simulink model "lab5"  (R2023b)
settings: Solver=ode4  StartTime=0.0  StopTime=100.0  FixedStep=2^(-6)  RelTol=1e-3
settings Model: Creator=insomnia  LastModifiedBy=insomnia

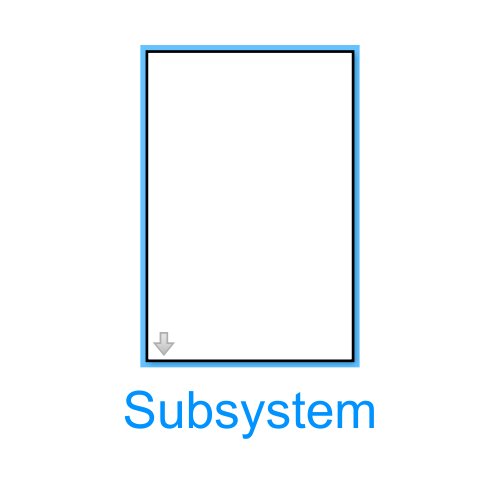
[thumbnail: Simulink's stored preview of the top-level diagram]
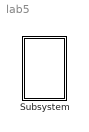
== system lab5 ==
  Subsystem : Subsystem  mask{g=9.81, l=2, m=3, k=5, r0=3, r1=1, th0=12, th1=6}

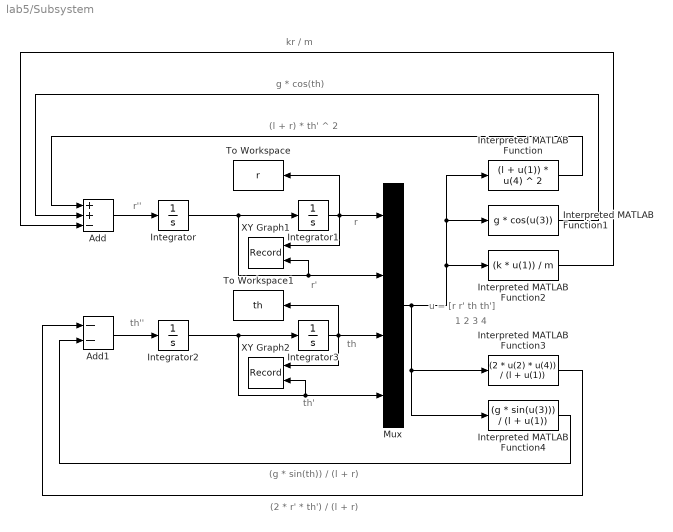
== system lab5/Subsystem ==
  note: (g * sin(th)) / (l + r)
  note: (2 * r' * th') / (l + r)
  note: th''
  note: r''
  note: kr / m
  note: g * cos(th)
  note: (l + r) * th' ^ 2
  note: th'
  note: th
  note: r'
  note: r
  note: 1 2 3 4
  note: u = [r r' th th']
  Add : Sum  Inputs=++-
  Add1 : Sum  Inputs=--
  Integrator : Integrator  InitialCondition=r1
  Integrator1 : Integrator  InitialCondition=r0
  Integrator2 : Integrator  InitialCondition=th1*pi/180
  Integrator3 : Integrator  InitialCondition=th0*pi/180
  Interpreted MATLAB Function : MATLABFcn  MATLABFcn=(l + u(1)) * u(4) ^ 2  OutputDimensions=1
  Interpreted MATLAB Function1 : MATLABFcn  MATLABFcn=g * cos(u(3))  OutputDimensions=1
  Interpreted MATLAB Function2 : MATLABFcn  MATLABFcn=(k * u(1)) / m  OutputDimensions=1
  Interpreted MATLAB Function3 : MATLABFcn  MATLABFcn=(2 * u(2) * u(4)) / (l + u(1))  OutputDimensions=1
  Interpreted MATLAB Function4 : MATLABFcn  MATLABFcn=(g * sin(u(3))) / (l + u(1))  OutputDimensions=1
  Mux : Mux
  To Workspace : ToWorkspace  VariableName=r  SampleTime=-1
  To Workspace1 : ToWorkspace  VariableName=th  SampleTime=-1
  XY Graph1 : Record  FileSettingsInternal="{\"entries\":[{\"content\":{\"excelSettings\":{\"content\":{},\"type\":\"Streamout.ExcelSettings\"}},\"type\":\"Streamout.FileSettingStorage\",\"uuid\":\"\"}],\"packageUris\":[\"http:\\/\\/schema.mathworks.com\\/mf0\\/streamout_blocks\\/R2020a\"],\"version\":\"1.0\"}"  Layout=[1 1]  SignalsInternal="{\"entries\":[{\"content\":{\"signals\":[{\"content\":{\"blockPath\":[],\"dimensions\":[1],\"domain\":\"\",\"lineColor\":\"#a2142f\",\"plots\":[ 1 ],\"port\":1,\"sid\":[\"\"],\"signalID\":1,\"signalName\":\"Integrator1\"},\"type\":\"RecordBlkView.Signal\",\"uuid\":\"\"},{\"content\":{\"blockPath\":[],\"dimensions\":[1],\"domain\":\"\",\"lineColor\":\"#139fff\",\"plots\":[ 1 ],\"port\":2,\"sid\":[\"\"],\"signalID\":2,\"signalName\":\"Integrator\"},\"type\":\"RecordBlkView.Signal\",\"uuid\":\"\"}]},\"type\":\"RecordBlkView.InputSignals\",\"uuid\":\"\"}],\"packageUris\":[\"http:\\/\\/schema.mathworks.com\\/mf0\\/streamout_blocks\\/R2020a\"],\"version\":\"1.0\"}"  VisualizationBindings="{\"xyplotplugin\":{\"info\":[{\"series\":[{\"bindingParametersList\":[{\"parameter\":\"X-Axis\",\"signalID\":1,\"signalName\":\"Integrator1\"},{\"parameter\":\"Y-Axis\",\"signalID\":2,\"signalName\":\"Integrator\"}],\"seriesID\":0}],\"subplotID\":1}]}}"  CompatibilityTag=XY
  XY Graph2 : Record  FileSettingsInternal="{\"entries\":[{\"content\":{\"excelSettings\":{\"content\":{},\"type\":\"Streamout.ExcelSettings\"}},\"type\":\"Streamout.FileSettingStorage\",\"uuid\":\"\"}],\"packageUris\":[\"http:\\/\\/schema.mathworks.com\\/mf0\\/streamout_blocks\\/R2020a\"],\"version\":\"1.0\"}"  Layout=[1 1]  SignalsInternal="{\"entries\":[{\"content\":{\"signals\":[{\"content\":{\"blockPath\":[],\"dimensions\":[1],\"domain\":\"\",\"lineColor\":\"#a2142f\",\"plots\":[ 1 ],\"port\":1,\"sid\":[\"\"],\"signalID\":1,\"signalName\":\"Integrator3\"},\"type\":\"RecordBlkView.Signal\",\"uuid\":\"\"},{\"content\":{\"blockPath\":[],\"dimensions\":[1],\"domain\":\"\",\"lineColor\":\"#139fff\",\"plots\":[ 1 ],\"port\":2,\"sid\":[\"\"],\"signalID\":2,\"signalName\":\"Integrator2\"},\"type\":\"RecordBlkView.Signal\",\"uuid\":\"\"}]},\"type\":\"RecordBlkView.InputSignals\",\"uuid\":\"\"}],\"packageUris\":[\"http:\\/\\/schema.mathworks.com\\/mf0\\/streamout_blocks\\/R2020a\"],\"version\":\"1.0\"}"  VisualizationBindings="{\"xyplotplugin\":{\"info\":[{\"series\":[{\"bindingParametersList\":[{\"parameter\":\"X-Axis\",\"signalID\":1,\"signalName\":\"Integrator3\"},{\"parameter\":\"Y-Axis\",\"signalID\":2,\"signalName\":\"Integrator2\"}],\"seriesID\":0}],\"subplotID\":1}]}}"  CompatibilityTag=XY
  wires:
  Interpreted MATLAB Function1/1 -> Add/2
  Mux/1 -> Interpreted MATLAB Function4/1, Interpreted MATLAB Function3/1, Interpreted MATLAB Function2/1, Interpreted MATLAB Function1/1, Interpreted MATLAB Function/1
  Interpreted MATLAB Function2/1 -> Add/3
  Integrator2/1 -> XY Graph2/2, Mux/4, Integrator3/1
  Integrator3/1 -> XY Graph2/1, To Workspace1/1, Mux/3
  Interpreted MATLAB Function4/1 -> Add1/2
  Integrator/1 -> XY Graph1/2, Mux/2, Integrator1/1
  Add/1 -> Integrator/1
  Add1/1 -> Integrator2/1
  Integrator1/1 -> To Workspace/1, XY Graph1/1, Mux/1
  Interpreted MATLAB Function3/1 -> Add1/1
  Interpreted MATLAB Function/1 -> Add/1
